simulink model "VannTankSemesterProsjekt"  (R2025a)
settings: Solver=VariableStepAuto  StartTime=0.0  StopTime=1000  RelTol=1e-3
libraries: slpidlib x1
settings Model: SimulationMode=accelerator  Creator=eirik  LastModifiedBy=eirik

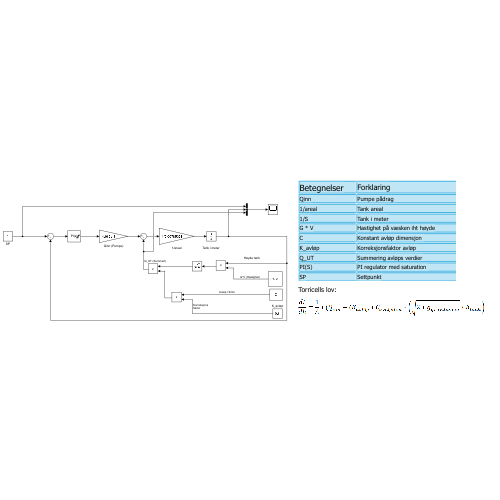
[thumbnail: Simulink's stored preview of the top-level diagram]
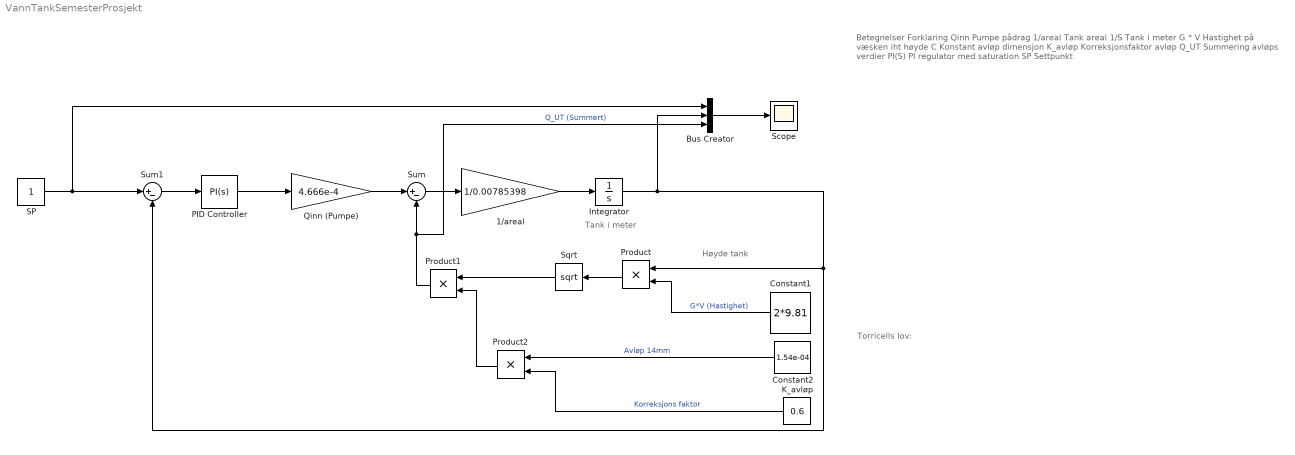
== system VannTankSemesterProsjekt ==
  note: Betegnelser
      | Forklaring
      |
      | Qinn
      | Pumpe pådrag
      |
      | 1/areal
      | Tank areal
      |
      | 1/S
      | Tank i meter
      |
      | G * V
      | Hastighet på væsken iht høyde
      |
      | C
      | Konstant avløp dimensjon
      |
      | K_avløp
      | Korreksjonsfaktor avløp
      |
      | Q_UT
      | Summering avløps verdier
      |
      | PI(S)
      | PI regulator med saturation
      |
      | SP
      | Settpunkt
  note: Torricells lov:
  note: Høyde tank
  note: Tank i meter
  1/areal : Gain  Gain=1/0.00785398
  Bus Creator : BusCreator  Inputs=3
  Constant1 : Constant  Value=2*9.81
  Constant2 : Constant  Value=1.54e-04
  Integrator : Integrator  InitialCondition=0.001
  K_avløp : Constant  Value=0.6
  PID Controller : slpidlib/PID Controller  Controller=PI  Form=Parallel  TimeDomain=Continuous-time  UseExternalTs=off  SampleTime=-1  IntegratorMethod=Forward Euler  FilterMethod=Forward Euler  ControllerParametersSource=internal  P=5  I=15  UseKiTs=off  D=0  UseExternalDerivativeSource=off  N=100  UseFilter=on  TunerSelectOption=Transfer Function Based (PID Tuner App)  InitialConditionSource=internal  InitialConditionForIntegrator=0  InitialConditionForFilter=0  DifferentiatorICPrevScaledInput=0  ExternalReset=none  TrackingMode=off  Kt=1  LimitOutput=on  SatLimitsSource=internal  UpperSaturationLimit=1  LowerSaturationLimit=0  LinearizeAsGain=off  AntiWindupMode=back-calculation  Kb=2  LimitIntegrator=off  UpperIntegratorSaturationLimit=inf  LowerIntegratorSaturationLimit=-inf  POutMin=[]  POutMax=[]  IOutMin=[]  IOutMax=[]  DOutMin=[]  DOutMax=[]  NOutMin=[]  NOutMax=[]  SumOutMin=[]  SumOutMax=[]  SaturationOutMin=[]  SaturationOutMax=[]  PParamMin=[]  PParamMax=[]  IParamMin=[]  IParamMax=[]  DParamMin=[]  DParamMax=[]  NParamMin=[]  NParamMax=[]  KbParamMin=[]  KbParamMax=[]  KtParamMin=[]  KtParamMax=[]  KbOutMin=[]  KbOutMax=[]  KtOutMin=[]  KtOutMax=[]  IntegratorOutMin=[]  IntegratorOutMax=[]  FilterOutMin=[]  FilterOutMax=[]  SumI1OutMin=[]  SumI1OutMax=[]  SumI2OutMin=[]  SumI2OutMax=[]  SumI3OutMin=[]  SumI3OutMax=[]  SumI4OutMin=[]  SumI4OutMax=[]  SumDOutMin=[]  SumDOutMax=[]  DifferentiatorOutMin=[]  DifferentiatorOutMax=[]  FilterDiffOutCoefMin=[]  FilterDiffOutCoefMax=[]  ReciprocalOutMin=[]  ReciprocalOutMax=[]  SumDenOutMin=[]  SumDenOutMax=[]  SumNumOutMin=[]  SumNumOutMax=[]  DivideOutMin=[]  DivideOutMax=[]  UdiffTsProdOutMin=[]  UdiffTsProdOutMax=[]  NTsProdOutMin=[]  NTsProdOutMax=[]  UintegralTsProdOutMin=[]  UintegralTsProdOutMax=[]  UngainTsProdOutMin=[]  UngainTsProdOutMax=[]  ClampingZeroOutDataTypeStr=Inherit: Inherit via back propagation  ClampingZeroOutMin=[]  ClampingZeroOutMax=[]  FilterDenConstantOutDataTypeStr=Inherit: Inherit via back propagation  FilterDenConstantOutMin=[]  FilterDenConstantOutMax=[]  PCopyOutDataTypeStr=Inherit: Inherit via back propagation  PCopyOutMin=[]  PCopyOutMax=[]  NCopyOutDataTypeStr=Inherit: Inherit via back propagation  NCopyOutMin=[]  NCopyOutMax=[]  IntegratorContinuousStateAttributes=''  IntegratorStateMustResolveToSignalObject=off  IntegratorRTWStateStorageClass=Auto  FilterContinuousStateAttributes=''  FilterStateMustResolveToSignalObject=off  FilterRTWStateStorageClass=Auto  ParallelPVariant=InternalParameters  IdealPVariant=Disabled  IVariant=InternalParameters  DVariant=Disabled  IntegratorVariant=Continuous  SatVariant=Enabled  AWVariant=BackCalculation  PCopyVariant=Disabled  TRVariant=Disabled  FdbkBlocksVariant=Forward  IdealPFdbkVariant=Disabled  SatFdbkVariant=Disabled  DerivativeFilterVariant=Disabled  NVariant=Disabled  NCopyVariant=Disabled_SignalSpec  FilterICVariant=Disabled  IntegratorICVariant=InternalICs  ExternalResetVariant=Disabled  TRSumVariant=Passthrough  SumFdbkVariant=Disabled  SumVariant=Sum_PI  TsampFilterVariant=InternalTs  TsampNgainVariant=Passthrough  TsampIntegralVariant=Disabled_SignalSpec  ExternalSaturationOutDataTypeStr=Inherit: Same as second input  DerivativeSourceVariant=Disabled  PreIntVariant=InternalPreInt
  Product : Product
  Product1 : Product
  Product2 : Product
  Qinn (Pumpe) : Gain  Gain=4.666e-4
  SP : Constant
  Scope : Scope
      settings: ActiveDisplayYMinimum=0.93990210773933036  ActiveDisplayYMaximum=1.0367026214781461
  Sqrt : Sqrt
  Sum : Sum  Inputs=|+-
  Sum1 : Sum  Inputs=|+-
  wires:
  Sum1/1 -> PID Controller/1
  Integrator/1 -> Bus Creator/2, Product/1, Sum1/2
  Sum/1 -> 1/areal/1
  1/areal/1 -> Integrator/1
  Qinn (Pumpe)/1 -> Sum/1
  PID Controller/1 -> Qinn (Pumpe)/1
  SP/1 -> Bus Creator/1, Sum1/1
  Constant1/1 -> Product/2  "G*V (Hastighet)"
  Product1/1 -> Bus Creator/3, Sum/2  "Q_UT (Summert)"
  Product/1 -> Sqrt/1
  Sqrt/1 -> Product1/1
  Constant2/1 -> Product2/1  "Avløp 14mm"
  K_avløp/1 -> Product2/2  "Korreksjons faktor"
  Product2/1 -> Product1/2
  Bus Creator/1 -> Scope/1
